simulink model "HyperscaleDataCenter"  (R2025b)
settings: Solver=VariableStepAuto  StartTime=0.0  StopTime=10  FixedStep=5e-5  RelTol=1e-4
PostLoadFcn:
  | HyperscaleDataCenterParam
values from neighbouring files (symbols this model uses):
  baseVoltageDC = 800    [DataCenterBBUParam.m]    (also in HyperscaleDataCenterParam.m; UPSBESSParam.m)
  bess_Ki = bess.controller.Ki    [SSTBESSParam.m]
  bess_Kp = bess.controller.Kp    [SSTBESSParam.m]
  droopGain = 0.02    [HyperscaleDataCenterParam.m]    (also in SSTBESSParam.m; UPSBESSParam.m)
  peakShavingPowerLimit = 800e3    (= 800000)    [HyperscaleDataCenterParam.m]
  powerTau = 0.005    [HyperscaleDataCenterParam.m]
  Prated_batt = 40e3    (= 40000)    [HyperscaleDataCenterParam.m]
  tauPS = 0.1    [HyperscaleDataCenterParam.m]
  Ts = 50e-6    (= 5e-05)    [BBUParam.m]    (also in DataCenterBBUParam.m; HyperscaleDataCenterParam.m)
  Ts_PS = 1e-3    (= 0.001)    [HyperscaleDataCenterParam.m]
undefined symbols (not defined in the file or in its folder): bbu, DiscIntNeverNeededParam, dspblkCoreblockFVToolHelper, ee_sli_rtmsupport, gcbh, grid, rack, sst, ups
libraries: fl_lib x80, nesl_utility x42, datacenter_lib x20, ee_lib x17, simulink x10, eeGeneralControl x9, slpidlib x6, microgridRenewables_lib x4, eeTransforms x4, batteryecm_lib x3, eeSinusoidalMeasurementV2 x2, simulink_extras x1
(part 5 of 5)

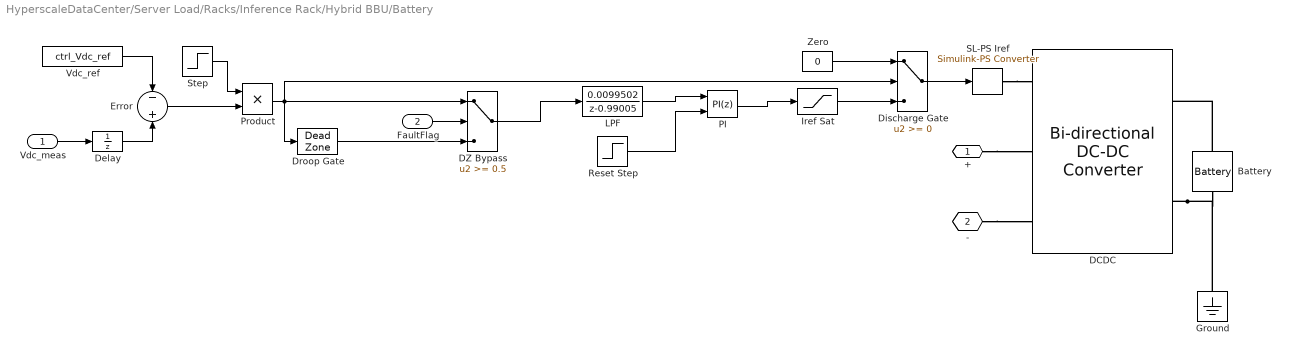
== system HyperscaleDataCenter/Server Load/Racks/Inference Rack/Hybrid BBU/Battery ==
  Vdc_meas : Inport
  FaultFlag : Inport  Port=2
  Battery : batteryecm_lib/Battery  Vnom=800 V  prm_dir=simscape.enum.battery.prm_dir.disabled  R1_dis=0.002 Ohm  R1_ch=0.002 Ohm  R1=0.004 Ohm  prm_AH=simscape.enum.battery.prm_AH.infinite  AH=50 A*hr  V1=11.5 V  AH1=25 A*hr  prm_R2=simscape.enum.battery.prm_R2.disabled  R2=2000 Ohm  Tmeas=298.15 K  charge_measurement_port=simscape.enum.battery.enable.no  prm_dyn=simscape.enum.battery.prm_dyn.off  Rp1=0.001 Ohm  tau1=30 s  Rp2=0.001 Ohm  tau2=30 s  Rp3=0.001 Ohm  tau3=30 s  Rp4=0.001 Ohm  tau4=30 s  Rp5=0.001 Ohm  tau5=30 s  prm_fade=simscape.enum.battery.prm_fade.disabled  N_fade=100  AH_fade=45 A*hr  R1_fade=2.02 Ohm  R1_ch_fade=2.02 Ohm  V1_fade=10.35 V  prm_age=simscape.enum.battery.prm_age.disabled  prm_age_OCV=simscape.enum.battery.prm_age_OCV.OCV  OCV_age=0.9  SOC_age=60  Tmeas_age=298.15 K  delta_time_age_vec=[0] d  temperature_age_vec=[273] K  OCV_scaling_age=2.2134e6  OCV_offset_age=1.632e6  temp_exp_age=0.515833569 V  t_exp_age=0.75  Vnom_T2=12 V  R1_T2=2.2 Ohm  R1_T2_dis=2.2 Ohm  R1_T2_ch=2.2 Ohm  V1_T2=11.4 V  R2_T2=2200 Ohm  Rp1_T2=0.005 Ohm  tau1_T2=30 s  Rp2_T2=0.005 Ohm  tau2_T2=30 s  Rp3_T2=0.005 Ohm  tau3_T2=30 s  Rp4_T2=0.005 Ohm  tau4_T2=30 s  Rp5_T2=0.005 Ohm  tau5_T2=30 s  Tmeas2=273.15 K  thermal_port=simscape.enum.thermaleffects.omit  thermal_mass=30000 J/K  i_specify=off  i_priority=None  i=0 A  i_nominal_specify=off  i_nominal_value=1  i_nominal_unit=A  v_specify=on  v_priority=None  v=800 V  v_nominal_specify=off  v_nominal_value=1  v_nominal_unit=V  charge_specify=off  charge_priority=None  charge=50 A*hr  charge_nominal_specify=off  charge_nominal_value=1  charge_nominal_unit=A*hr  num_cycles_specify=off  num_cycles_priority=High  num_cycles=0  num_cycles_nominal_specify=off  num_cycles_nominal_value=1  num_cycles_nominal_unit=1  temperature_specify=off  temperature_priority=High  temperature=298.15 K  temperature_nominal_specify=off  temperature_nominal_value=1  temperature_nominal_unit=K
  DCDC : microgridRenewables_lib/Bi-directional DC-DC Converter  efficiency_option=ee.enum.converters.efficiency.constant  efficiency_fixed=100  i_vec=[0, 2, 5] A  efficiency_vec=[90, 95, 98]  iL_specify=off  iL_priority=High  iL=0 A  iL_nominal_specify=off  iL_nominal_value=1  iL_nominal_unit=A  vc_specify=off  vc_priority=High  vc=0 V  vc_nominal_specify=off  vc_nominal_value=1  vc_nominal_unit=V  i1_specify=on  i1_priority=Low  i1=0 A  i1_nominal_specify=off  i1_nominal_value=1  i1_nominal_unit=A  i2_specify=on  i2_priority=Low  i2=0 A  i2_nominal_specify=off  i2_nominal_value=1  i2_nominal_unit=A  v1_specify=off  v1_priority=None  v1=0 V  v1_nominal_specify=off  v1_nominal_value=1  v1_nominal_unit=V  v2_specify=off  v2_priority=High  v2=800 V  v2_nominal_specify=off  v2_nominal_value=1  v2_nominal_unit=V
      settings: InternalSimscapePortConfiguration="{\"Bottom\":[],\"Left\":[{\"id\":\"Iref\",\"label\":\"Iref\",\"type\":\"input\"},{\"id\":\"p1\",\"label\":\"1+\",\"type\":\"foundation.electrical.electrical\"},{\"id\":\"n1\",\"label\":\"1-\",\"type\":\"foundation.electrical.electrical\"}],\"Right\":[{\"id\":\"p2\",\"label\":\"2+\",\"type\":\"foundation.electrical.electrical\"},{\"id\":\"n2\",\"label\":\"2-\",\"type\":\"foundation.electrical.electrical\"}],\"Top\":[]}"
  DZ Bypass : Switch  Threshold=0.5  SaturateOnIntegerOverflow=off  InputSameDT=off
  Delay : UnitDelay  InitialCondition=800  SampleTime=ctrl_Ts
  Discharge Gate : Switch  SaturateOnIntegerOverflow=off  InputSameDT=off
  Droop Gate : DeadZone  LowerValue=-60  UpperValue=60
  Error : Sum  Inputs=-+
  Ground : fl_lib/Electrical/Electrical Elements/Electrical Reference
  Iref Sat : Saturate  UpperLimit=0  LowerLimit=-10000
  LPF : DiscreteTransferFcn  Numerator=[0.0099502]  Denominator=[1 -0.99005]
  PI : slpidlib/PID Controller  Controller=PI  Form=Parallel  TimeDomain=Discrete-time  UseExternalTs=off  SampleTime=ctrl_Ts  IntegratorMethod=Forward Euler  FilterMethod=Forward Euler  ControllerParametersSource=internal  P=batt_Kp_ctrl  I=batt_Ki_ctrl  UseKiTs=off  D=0  UseExternalDerivativeSource=off  N=100  UseFilter=on  TunerSelectOption=Transfer Function Based (PID Tuner App)  InitialConditionSource=internal  InitialConditionForIntegrator=0  InitialConditionForFilter=0  DifferentiatorICPrevScaledInput=0  ExternalReset=rising  TrackingMode=off  Kt=1  LimitOutput=on  SatLimitsSource=internal  UpperSaturationLimit=0  LowerSaturationLimit=-batt_Imax  LinearizeAsGain=off  AntiWindupMode=clamping  Kb=1  LimitIntegrator=off  UpperIntegratorSaturationLimit=inf  LowerIntegratorSaturationLimit=-inf  POutMin=[]  POutMax=[]  IOutMin=[]  IOutMax=[]  DOutMin=[]  DOutMax=[]  NOutMin=[]  NOutMax=[]  SumOutMin=[]  SumOutMax=[]  SaturationOutMin=[]  SaturationOutMax=[]  PParamMin=[]  PParamMax=[]  IParamMin=[]  IParamMax=[]  DParamMin=[]  DParamMax=[]  NParamMin=[]  NParamMax=[]  KbParamMin=[]  KbParamMax=[]  KtParamMin=[]  KtParamMax=[]  KbOutMin=[]  KbOutMax=[]  KtOutMin=[]  KtOutMax=[]  IntegratorOutMin=[]  IntegratorOutMax=[]  FilterOutMin=[]  FilterOutMax=[]  SumI1OutMin=[]  SumI1OutMax=[]  SumI2OutMin=[]  SumI2OutMax=[]  SumI3OutMin=[]  SumI3OutMax=[]  SumI4OutMin=[]  SumI4OutMax=[]  SumDOutMin=[]  SumDOutMax=[]  DifferentiatorOutMin=[]  DifferentiatorOutMax=[]  FilterDiffOutCoefMin=[]  FilterDiffOutCoefMax=[]  ReciprocalOutMin=[]  ReciprocalOutMax=[]  SumDenOutMin=[]  SumDenOutMax=[]  SumNumOutMin=[]  SumNumOutMax=[]  DivideOutMin=[]  DivideOutMax=[]  UdiffTsProdOutMin=[]  UdiffTsProdOutMax=[]  NTsProdOutMin=[]  NTsProdOutMax=[]  UintegralTsProdOutMin=[]  UintegralTsProdOutMax=[]  UngainTsProdOutMin=[]  UngainTsProdOutMax=[]  ClampingZeroOutDataTypeStr=Inherit: Inherit via back propagation  ClampingZeroOutMin=[]  ClampingZeroOutMax=[]  FilterDenConstantOutDataTypeStr=Inherit: Inherit via back propagation  FilterDenConstantOutMin=[]  FilterDenConstantOutMax=[]  PCopyOutDataTypeStr=Inherit: Inherit via back propagation  PCopyOutMin=[]  PCopyOutMax=[]  NCopyOutDataTypeStr=Inherit: Inherit via back propagation  NCopyOutMin=[]  NCopyOutMax=[]  IntegratorContinuousStateAttributes=''  IntegratorStateMustResolveToSignalObject=off  IntegratorRTWStateStorageClass=Auto  FilterContinuousStateAttributes=''  FilterStateMustResolveToSignalObject=off  FilterRTWStateStorageClass=Auto  ParallelPVariant=InternalParameters  IdealPVariant=Disabled  IVariant=InternalParameters  DVariant=Disabled  IntegratorVariant=Discrete  SatVariant=Enabled  AWVariant=DiscClampingParallel  PCopyVariant=Disabled  TRVariant=Disabled  FdbkBlocksVariant=Forward  IdealPFdbkVariant=Disabled  SatFdbkVariant=Disabled  DerivativeFilterVariant=Disabled  NVariant=Disabled  NCopyVariant=Disabled_SignalSpec  FilterICVariant=Disabled  IntegratorICVariant=InternalICs  ExternalResetVariant=ExternalReset  TRSumVariant=Passthrough  SumFdbkVariant=Disabled  SumVariant=Sum_PI  TsampFilterVariant=InternalTs  TsampNgainVariant=Passthrough  TsampIntegralVariant=Disabled_SignalSpec  ExternalSaturationOutDataTypeStr=Inherit: Same as second input  DerivativeSourceVariant=Disabled  PreIntVariant=InternalPreInt
      settings: LibrarySourceBlock=simulink/Discrete/Discrete PID Controller
  Product : Product
  Reset Step : Step  Time=0.5  SampleTime=0
  SL-PS Iref : nesl_utility/Simulink-PS Converter  PhysicalDomain=network_engine_domain  SubClassName=ps_input  LeftPortType=input  RightPortType=output  PseudoPeriodic=off  Frequencies=[]  NoiseDistribution=none  NoiseParameters=[]  Unit=1  AffineConversion=off  FilteringAndDerivatives=filter  SimscapeFilterOrder=1  InputFilterTimeConstant=5e-05  UdotUserProvided=0
  Step : Step  Time=0  SampleTime=0
  Vdc_ref : Constant  Value=ctrl_Vdc_ref
  Zero : Constant  Value=0
  + : PMIOPort  Side=Left
  - : PMIOPort  Port=2  Side=Left
  wires:
  Vdc_ref/1 -> Error/1
  Delay/1 -> Error/2
  LPF/1 -> PI/1
  PI/1 -> Iref Sat/1
  Vdc_meas/1 -> Delay/1
  FaultFlag/1 -> DZ Bypass/2
  Droop Gate/1 -> DZ Bypass/3
  DZ Bypass/1 -> LPF/1
  Zero/1 -> Discharge Gate/1
  Iref Sat/1 -> Discharge Gate/3
  Discharge Gate/1 -> SL-PS Iref/1
  Step/1 -> Product/1
  Error/1 -> Product/2
  Product/1 -> Discharge Gate/2, Droop Gate/1, DZ Bypass/1
  Reset Step/1 -> PI/2
  connections:
  +/RConn1 -- DCDC/LConn2
  DCDC/RConn2 -- Ground/LConn1 -- Battery/RConn1
  Battery/LConn1 -- DCDC/RConn1
  -/RConn1 -- DCDC/LConn3
  SL-PS Iref/RConn1 -- DCDC/LConn1

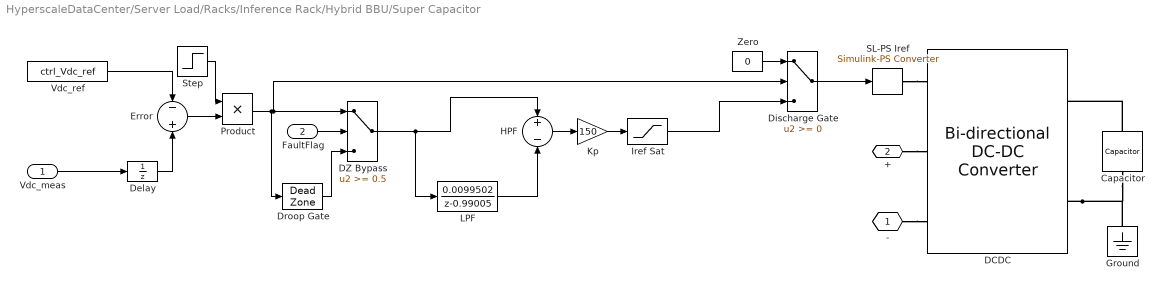
== system HyperscaleDataCenter/Server Load/Racks/Inference Rack/Hybrid BBU/Super Capacitor ==
  Vdc_meas : Inport
  FaultFlag : Inport  Port=2
  Capacitor : fl_lib/Electrical/Electrical Elements/Capacitor  c=5 F  r=1e-06 Ohm  g=0 1/Ohm  i_specify=off  i_priority=None  i=0 A  i_nominal_specify=off  i_nominal_value=1  i_nominal_unit=A  v_specify=on  v_priority=None  v=800 V  v_nominal_specify=off  v_nominal_value=1  v_nominal_unit=V  vc_specify=on  vc_priority=None  vc=800 V  vc_nominal_specify=off  vc_nominal_value=1  vc_nominal_unit=V
  DCDC : microgridRenewables_lib/Bi-directional DC-DC Converter  efficiency_option=ee.enum.converters.efficiency.constant  efficiency_fixed=100  i_vec=[0, 2, 5] A  efficiency_vec=[90, 95, 98]  iL_specify=off  iL_priority=High  iL=0 A  iL_nominal_specify=off  iL_nominal_value=1  iL_nominal_unit=A  vc_specify=off  vc_priority=High  vc=0 V  vc_nominal_specify=off  vc_nominal_value=1  vc_nominal_unit=V  i1_specify=on  i1_priority=Low  i1=0 A  i1_nominal_specify=off  i1_nominal_value=1  i1_nominal_unit=A  i2_specify=on  i2_priority=Low  i2=0 A  i2_nominal_specify=off  i2_nominal_value=1  i2_nominal_unit=A  v1_specify=off  v1_priority=None  v1=0 V  v1_nominal_specify=off  v1_nominal_value=1  v1_nominal_unit=V  v2_specify=off  v2_priority=High  v2=800 V  v2_nominal_specify=off  v2_nominal_value=1  v2_nominal_unit=V
      settings: InternalSimscapePortConfiguration="{\"Bottom\":[],\"Left\":[{\"id\":\"Iref\",\"label\":\"Iref\",\"type\":\"input\"},{\"id\":\"p1\",\"label\":\"1+\",\"type\":\"foundation.electrical.electrical\"},{\"id\":\"n1\",\"label\":\"1-\",\"type\":\"foundation.electrical.electrical\"}],\"Right\":[{\"id\":\"p2\",\"label\":\"2+\",\"type\":\"foundation.electrical.electrical\"},{\"id\":\"n2\",\"label\":\"2-\",\"type\":\"foundation.electrical.electrical\"}],\"Top\":[]}"
  DZ Bypass : Switch  Threshold=0.5  SaturateOnIntegerOverflow=off  InputSameDT=off
  Delay : UnitDelay  InitialCondition=800  SampleTime=ctrl_Ts
  Discharge Gate : Switch  SaturateOnIntegerOverflow=off  InputSameDT=off
  Droop Gate : DeadZone  LowerValue=-60  UpperValue=60
  Error : Sum  Inputs=-+
  Ground : fl_lib/Electrical/Electrical Elements/Electrical Reference
  HPF : Sum  Inputs=+-
  Iref Sat : Saturate  UpperLimit=0  LowerLimit=-12000
  Kp : Gain  Gain=150
  LPF : DiscreteTransferFcn  LoadFcn=dspblkCoreblockFVToolHelper(gcbh,'load');  Numerator=[0.0099502]  Denominator=[1 -0.99005]
      settings: CopyFcn=dspblkCoreblockFVToolHelper(gcbh,'copy');  DeleteFcn=dspblkCoreblockFVToolHelper(gcbh,'close');  ModelCloseFcn=dspblkCoreblockFVToolHelper(gcbh,'close');  PreSaveFcn=dspblkCoreblockFVToolHelper(gcbh,'presave');  PostSaveFcn=dspblkCoreblockFVToolHelper(gcbh,'postsave');  CloseFcn=dspblkCoreblockFVToolHelper(gcbh,'close');
  Product : Product
  SL-PS Iref : nesl_utility/Simulink-PS Converter  PhysicalDomain=network_engine_domain  SubClassName=ps_input  LeftPortType=input  RightPortType=output  PseudoPeriodic=off  Frequencies=[]  NoiseDistribution=none  NoiseParameters=[]  Unit=1  AffineConversion=off  FilteringAndDerivatives=filter  SimscapeFilterOrder=1  InputFilterTimeConstant=1e-05  UdotUserProvided=0
  Step : Step  Time=0  SampleTime=0
  Vdc_ref : Constant  Value=ctrl_Vdc_ref
  Zero : Constant  Value=0
  - : PMIOPort  Side=Left
  + : PMIOPort  Port=2  Side=Left
  wires:
  Vdc_ref/1 -> Error/1
  Delay/1 -> Error/2
  Kp/1 -> Iref Sat/1
  Droop Gate/1 -> DZ Bypass/3
  LPF/1 -> HPF/2
  HPF/1 -> Kp/1
  Vdc_meas/1 -> Delay/1
  FaultFlag/1 -> DZ Bypass/2
  DZ Bypass/1 -> HPF/1, LPF/1
  Zero/1 -> Discharge Gate/1
  Iref Sat/1 -> Discharge Gate/3
  Discharge Gate/1 -> SL-PS Iref/1
  Step/1 -> Product/1
  Error/1 -> Product/2
  Product/1 -> Droop Gate/1, Discharge Gate/2, DZ Bypass/1
  connections:
  +/RConn1 -- DCDC/LConn2
  DCDC/RConn2 -- Ground/LConn1 -- Capacitor/RConn1
  Capacitor/LConn1 -- DCDC/RConn1
  -/RConn1 -- DCDC/LConn3
  SL-PS Iref/RConn1 -- DCDC/LConn1

== system HyperscaleDataCenter/Server Load/Racks/Inference Rack/PDU Racks/Server Tray ==
  AmbCPU : fl_lib/Thermal/Thermal Elements/Convective Heat Transfer  thermal_type=foundation.enum.constant_variable.constant  area=cpuSurfArea*nCPU m^2  heat_tr_coeff=htc W/(K*m^2)  min_heat_tr_coeff=1e-3 W/(K*m^2)  T_specify=off  T_priority=None  T=0 K  T_nominal_specify=off  T_nominal_value=1  T_nominal_unit=K  Q_specify=off  Q_priority=None  Q=0 W  Q_nominal_specify=off  Q_nominal_value=1  Q_nominal_unit=W
  AmbGPU : fl_lib/Thermal/Thermal Elements/Convective Heat Transfer  thermal_type=foundation.enum.constant_variable.constant  area=gpuSurfArea*nGPU m^2  heat_tr_coeff=htc W/(K*m^2)  min_heat_tr_coeff=1e-3 W/(K*m^2)  T_specify=off  T_priority=None  T=0 K  T_nominal_specify=off  T_nominal_value=1  T_nominal_unit=K  Q_specify=off  Q_priority=None  Q=0 W  Q_nominal_specify=off  Q_nominal_value=1  Q_nominal_unit=W
  PS Add : fl_lib/Physical Signals/Functions/PS Add
  Server Chip CPU : datacenter_lib/Server Chip  processorType=ProcessorType.CPU  numGPUs=4  numCPUs=nCPU  gpuTDP=1200 W  gpuIdlePower=300 W  gpuPowerExponent=1.4  hbmPowPerGPU=80 W  hbmUtilizationFrac=0.7  cpuTDP=cpuTDPperSocket W  cpuIdlePower=cpuIdlePower W  cpuPowerExponent=cpuExponent  PleakageCoeff=cpuLeakage W/K  chipTnominal=cpuNominalDieT K  chipCth=cpuDieThermalC J/K  T_specify=on  T_priority=None  T=initialT K  T_nominal_specify=off  T_nominal_value=1  T_nominal_unit=K  Q_specify=off  Q_priority=None  Q=0 W  Q_nominal_specify=off  Q_nominal_value=1  Q_nominal_unit=W
      settings: InternalSimscapePortConfiguration="{\"Bottom\":[{\"id\":\"H\",\"label\":\"H\",\"type\":\"foundation.thermal.thermal\"}],\"Left\":[{\"id\":\"U\",\"label\":\"U\",\"type\":\"input\"}],\"Right\":[{\"id\":\"Pow\",\"label\":\"P\",\"type\":\"output\"},{\"id\":\"Tchip\",\"label\":\"T\",\"type\":\"output\"}],\"Top\":[]}"
  Server Chip GPU : datacenter_lib/Server Chip  processorType=ProcessorType.GPU  numGPUs=nGPU  numCPUs=nCPU  gpuTDP=gpuTDPperDie W  gpuIdlePower=gpuIdlePower W  gpuPowerExponent=gpuExponent  hbmPowPerGPU=gpuHBMpower W  hbmUtilizationFrac=gpuHBMutil  cpuTDP=cpuTDPperSocket W  cpuIdlePower=cpuIdlePower W  cpuPowerExponent=1.1  PleakageCoeff=gpuLeakage W/K  chipTnominal=gpuNominalDieT K  chipCth=gpuDieThermalC J/K  T_specify=on  T_priority=None  T=initialT K  T_nominal_specify=off  T_nominal_value=1  T_nominal_unit=K  Q_specify=off  Q_priority=None  Q=0 W  Q_nominal_specify=off  Q_nominal_value=1  Q_nominal_unit=W
      settings: InternalSimscapePortConfiguration="{\"Bottom\":[{\"id\":\"H\",\"label\":\"H\",\"type\":\"foundation.thermal.thermal\"}],\"Left\":[{\"id\":\"U\",\"label\":\"U\",\"type\":\"input\"}],\"Right\":[{\"id\":\"Pow\",\"label\":\"P\",\"type\":\"output\"},{\"id\":\"Tchip\",\"label\":\"T\",\"type\":\"output\"}],\"Top\":[]}"
  TR_CPU_Amb : fl_lib/Thermal/Thermal Elements/Thermal Resistance  resistance=cpuAmbientR/nGPU K/W  T_specify=off  T_priority=None  T=0 K  T_nominal_specify=off  T_nominal_value=1  T_nominal_unit=K  Q_specify=off  Q_priority=None  Q=0 W  Q_nominal_specify=off  Q_nominal_value=1  Q_nominal_unit=W
  TR_CPU_substrate : fl_lib/Thermal/Thermal Elements/Thermal Resistance  resistance=cpuHeatSinkR/nGPU K/W  T_specify=off  T_priority=None  T=0 K  T_nominal_specify=off  T_nominal_value=1  T_nominal_unit=K  Q_specify=off  Q_priority=None  Q=0 W  Q_nominal_specify=off  Q_nominal_value=1  Q_nominal_unit=W
  TR_GPU_Amb : fl_lib/Thermal/Thermal Elements/Thermal Resistance  resistance=gpuAmbientR/nGPU K/W  T_specify=off  T_priority=None  T=0 K  T_nominal_specify=off  T_nominal_value=1  T_nominal_unit=K  Q_specify=off  Q_priority=None  Q=0 W  Q_nominal_specify=off  Q_nominal_value=1  Q_nominal_unit=W
  TR_GPU_substrate : fl_lib/Thermal/Thermal Elements/Thermal Resistance  resistance=gpuHeatSinkR/nGPU K/W  T_specify=off  T_priority=None  T=0 K  T_nominal_specify=off  T_nominal_value=1  T_nominal_unit=K  Q_specify=off  Q_priority=None  Q=0 W  Q_nominal_specify=off  Q_nominal_value=1  Q_nominal_unit=W
  TR_Tray_Amb : fl_lib/Thermal/Thermal Elements/Thermal Resistance  resistance=trayThermalR K/W  T_specify=off  T_priority=None  T=0 K  T_nominal_specify=off  T_nominal_value=1  T_nominal_unit=K  Q_specify=off  Q_priority=None  Q=0 W  Q_nominal_specify=off  Q_nominal_value=1  Q_nominal_unit=W
  Tray Thermal Mass : fl_lib/Thermal/Thermal Elements/Thermal Mass  mass_type=foundation.enum.constant_variable.constant  mass=trayMass kg  sp_heat=trayCp J/(K*kg)  mass_min=1e-6 kg  num_ports=foundation.enum.numPorts2.two  m_specify=off  m_priority=None  m=1 kg  m_nominal_specify=off  m_nominal_value=1  m_nominal_unit=kg  T_specify=on  T_priority=None  T=initialT K  T_nominal_specify=off  T_nominal_value=1  T_nominal_unit=K  Q_specify=off  Q_priority=None  Q=0 W  Q_nominal_specify=off  Q_nominal_value=1  Q_nominal_unit=W
      settings: InternalSimscapePortConfiguration="{\"Bottom\":[],\"Left\":[{\"id\":\"M\",\"label\":\"\",\"type\":\"foundation.thermal.thermal\"}],\"Right\":[{\"id\":\"N\",\"label\":\"\",\"type\":\"foundation.thermal.thermal\"}],\"Top\":[]}"
  U_gpu : PMIOPort  Side=Left
  U_cpu : PMIOPort  Port=2  Side=Left
  P : PMIOPort  Port=3  Side=Right
  T_gpu : PMIOPort  Port=4  Side=Right
  T_cpu : PMIOPort  Port=5  Side=Right
  Hc : PMIOPort  Port=6  Side=Right
  Ha : PMIOPort  Port=7  Side=Left
  connections:
  AmbCPU/LConn1 -- TR_CPU_Amb/RConn1
  PS Add/LConn2 -- Server Chip CPU/RConn1
  PS Add/LConn1 -- Server Chip GPU/RConn1
  P/RConn1 -- PS Add/RConn1
  Ha/RConn1 -- AmbGPU/RConn1 -- AmbCPU/RConn1
  AmbGPU/LConn1 -- TR_GPU_Amb/LConn1
  TR_Tray_Amb/RConn1 -- Hc/RConn1
  Server Chip CPU/RConn2 -- T_cpu/RConn1
  Server Chip CPU/LConn1 -- U_cpu/RConn1
  Server Chip GPU/LConn1 -- U_gpu/RConn1
  TR_Tray_Amb/LConn1 -- Tray Thermal Mass/RConn1
  TR_GPU_substrate/LConn1 -- Server Chip GPU/RConn3 -- TR_GPU_Amb/RConn1
  Server Chip CPU/RConn3 -- TR_CPU_Amb/LConn1 -- TR_CPU_substrate/LConn1
  Server Chip GPU/RConn2 -- T_gpu/RConn1
  TR_CPU_substrate/RConn1 -- TR_GPU_substrate/RConn1 -- Tray Thermal Mass/LConn1

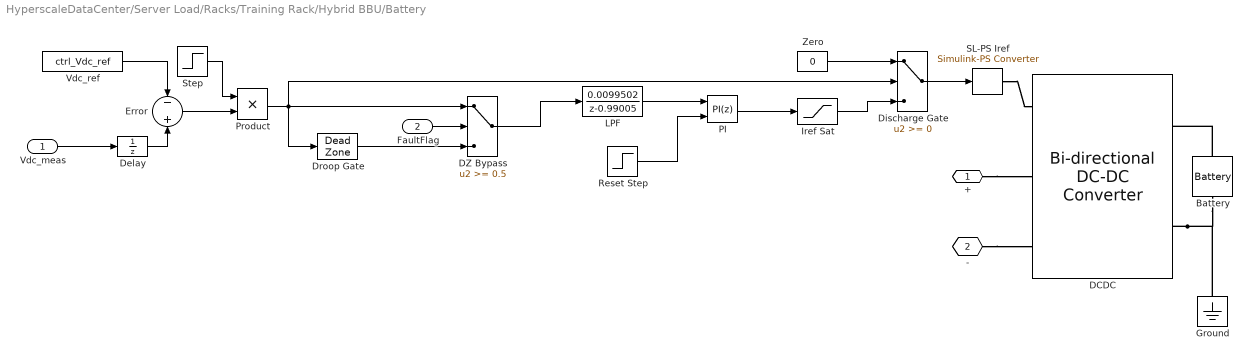
== system HyperscaleDataCenter/Server Load/Racks/Training Rack/Hybrid BBU/Battery ==
  Vdc_meas : Inport
  FaultFlag : Inport  Port=2
  Battery : batteryecm_lib/Battery  Vnom=800 V  prm_dir=simscape.enum.battery.prm_dir.disabled  R1_dis=0.002 Ohm  R1_ch=0.002 Ohm  R1=0.004 Ohm  prm_AH=simscape.enum.battery.prm_AH.infinite  AH=50 A*hr  V1=11.5 V  AH1=25 A*hr  prm_R2=simscape.enum.battery.prm_R2.disabled  R2=2000 Ohm  Tmeas=298.15 K  charge_measurement_port=simscape.enum.battery.enable.no  prm_dyn=simscape.enum.battery.prm_dyn.off  Rp1=0.001 Ohm  tau1=30 s  Rp2=0.001 Ohm  tau2=30 s  Rp3=0.001 Ohm  tau3=30 s  Rp4=0.001 Ohm  tau4=30 s  Rp5=0.001 Ohm  tau5=30 s  prm_fade=simscape.enum.battery.prm_fade.disabled  N_fade=100  AH_fade=45 A*hr  R1_fade=2.02 Ohm  R1_ch_fade=2.02 Ohm  V1_fade=10.35 V  prm_age=simscape.enum.battery.prm_age.disabled  prm_age_OCV=simscape.enum.battery.prm_age_OCV.OCV  OCV_age=0.9  SOC_age=60  Tmeas_age=298.15 K  delta_time_age_vec=[0] d  temperature_age_vec=[273] K  OCV_scaling_age=2.2134e6  OCV_offset_age=1.632e6  temp_exp_age=0.515833569 V  t_exp_age=0.75  Vnom_T2=12 V  R1_T2=2.2 Ohm  R1_T2_dis=2.2 Ohm  R1_T2_ch=2.2 Ohm  V1_T2=11.4 V  R2_T2=2200 Ohm  Rp1_T2=0.005 Ohm  tau1_T2=30 s  Rp2_T2=0.005 Ohm  tau2_T2=30 s  Rp3_T2=0.005 Ohm  tau3_T2=30 s  Rp4_T2=0.005 Ohm  tau4_T2=30 s  Rp5_T2=0.005 Ohm  tau5_T2=30 s  Tmeas2=273.15 K  thermal_port=simscape.enum.thermaleffects.omit  thermal_mass=30000 J/K  i_specify=off  i_priority=None  i=0 A  i_nominal_specify=off  i_nominal_value=1  i_nominal_unit=A  v_specify=on  v_priority=None  v=800 V  v_nominal_specify=off  v_nominal_value=1  v_nominal_unit=V  charge_specify=off  charge_priority=None  charge=50 A*hr  charge_nominal_specify=off  charge_nominal_value=1  charge_nominal_unit=A*hr  num_cycles_specify=off  num_cycles_priority=High  num_cycles=0  num_cycles_nominal_specify=off  num_cycles_nominal_value=1  num_cycles_nominal_unit=1  temperature_specify=off  temperature_priority=High  temperature=298.15 K  temperature_nominal_specify=off  temperature_nominal_value=1  temperature_nominal_unit=K
  DCDC : microgridRenewables_lib/Bi-directional DC-DC Converter  efficiency_option=ee.enum.converters.efficiency.constant  efficiency_fixed=100  i_vec=[0, 2, 5] A  efficiency_vec=[90, 95, 98]  iL_specify=off  iL_priority=High  iL=0 A  iL_nominal_specify=off  iL_nominal_value=1  iL_nominal_unit=A  vc_specify=off  vc_priority=High  vc=0 V  vc_nominal_specify=off  vc_nominal_value=1  vc_nominal_unit=V  i1_specify=on  i1_priority=Low  i1=0 A  i1_nominal_specify=off  i1_nominal_value=1  i1_nominal_unit=A  i2_specify=on  i2_priority=Low  i2=0 A  i2_nominal_specify=off  i2_nominal_value=1  i2_nominal_unit=A  v1_specify=off  v1_priority=None  v1=0 V  v1_nominal_specify=off  v1_nominal_value=1  v1_nominal_unit=V  v2_specify=off  v2_priority=High  v2=800 V  v2_nominal_specify=off  v2_nominal_value=1  v2_nominal_unit=V
      settings: InternalSimscapePortConfiguration="{\"Bottom\":[],\"Left\":[{\"id\":\"Iref\",\"label\":\"Iref\",\"type\":\"input\"},{\"id\":\"p1\",\"label\":\"1+\",\"type\":\"foundation.electrical.electrical\"},{\"id\":\"n1\",\"label\":\"1-\",\"type\":\"foundation.electrical.electrical\"}],\"Right\":[{\"id\":\"p2\",\"label\":\"2+\",\"type\":\"foundation.electrical.electrical\"},{\"id\":\"n2\",\"label\":\"2-\",\"type\":\"foundation.electrical.electrical\"}],\"Top\":[]}"
  DZ Bypass : Switch  Threshold=0.5  SaturateOnIntegerOverflow=off  InputSameDT=off
  Delay : UnitDelay  InitialCondition=800  SampleTime=ctrl_Ts
  Discharge Gate : Switch  SaturateOnIntegerOverflow=off  InputSameDT=off
  Droop Gate : DeadZone  LowerValue=-60  UpperValue=60
  Error : Sum  Inputs=-+
  Ground : fl_lib/Electrical/Electrical Elements/Electrical Reference
  Iref Sat : Saturate  UpperLimit=0  LowerLimit=-10000
  LPF : DiscreteTransferFcn  Numerator=[0.0099502]  Denominator=[1 -0.99005]
  PI : slpidlib/PID Controller  Controller=PI  Form=Parallel  TimeDomain=Discrete-time  UseExternalTs=off  SampleTime=ctrl_Ts  IntegratorMethod=Forward Euler  FilterMethod=Forward Euler  ControllerParametersSource=internal  P=batt_Kp_ctrl  I=batt_Ki_ctrl  UseKiTs=off  D=0  UseExternalDerivativeSource=off  N=100  UseFilter=on  TunerSelectOption=Transfer Function Based (PID Tuner App)  InitialConditionSource=internal  InitialConditionForIntegrator=0  InitialConditionForFilter=0  DifferentiatorICPrevScaledInput=0  ExternalReset=rising  TrackingMode=off  Kt=1  LimitOutput=on  SatLimitsSource=internal  UpperSaturationLimit=0  LowerSaturationLimit=-batt_Imax  LinearizeAsGain=off  AntiWindupMode=clamping  Kb=1  LimitIntegrator=off  UpperIntegratorSaturationLimit=inf  LowerIntegratorSaturationLimit=-inf  POutMin=[]  POutMax=[]  IOutMin=[]  IOutMax=[]  DOutMin=[]  DOutMax=[]  NOutMin=[]  NOutMax=[]  SumOutMin=[]  SumOutMax=[]  SaturationOutMin=[]  SaturationOutMax=[]  PParamMin=[]  PParamMax=[]  IParamMin=[]  IParamMax=[]  DParamMin=[]  DParamMax=[]  NParamMin=[]  NParamMax=[]  KbParamMin=[]  KbParamMax=[]  KtParamMin=[]  KtParamMax=[]  KbOutMin=[]  KbOutMax=[]  KtOutMin=[]  KtOutMax=[]  IntegratorOutMin=[]  IntegratorOutMax=[]  FilterOutMin=[]  FilterOutMax=[]  SumI1OutMin=[]  SumI1OutMax=[]  SumI2OutMin=[]  SumI2OutMax=[]  SumI3OutMin=[]  SumI3OutMax=[]  SumI4OutMin=[]  SumI4OutMax=[]  SumDOutMin=[]  SumDOutMax=[]  DifferentiatorOutMin=[]  DifferentiatorOutMax=[]  FilterDiffOutCoefMin=[]  FilterDiffOutCoefMax=[]  ReciprocalOutMin=[]  ReciprocalOutMax=[]  SumDenOutMin=[]  SumDenOutMax=[]  SumNumOutMin=[]  SumNumOutMax=[]  DivideOutMin=[]  DivideOutMax=[]  UdiffTsProdOutMin=[]  UdiffTsProdOutMax=[]  NTsProdOutMin=[]  NTsProdOutMax=[]  UintegralTsProdOutMin=[]  UintegralTsProdOutMax=[]  UngainTsProdOutMin=[]  UngainTsProdOutMax=[]  ClampingZeroOutDataTypeStr=Inherit: Inherit via back propagation  ClampingZeroOutMin=[]  ClampingZeroOutMax=[]  FilterDenConstantOutDataTypeStr=Inherit: Inherit via back propagation  FilterDenConstantOutMin=[]  FilterDenConstantOutMax=[]  PCopyOutDataTypeStr=Inherit: Inherit via back propagation  PCopyOutMin=[]  PCopyOutMax=[]  NCopyOutDataTypeStr=Inherit: Inherit via back propagation  NCopyOutMin=[]  NCopyOutMax=[]  IntegratorContinuousStateAttributes=''  IntegratorStateMustResolveToSignalObject=off  IntegratorRTWStateStorageClass=Auto  FilterContinuousStateAttributes=''  FilterStateMustResolveToSignalObject=off  FilterRTWStateStorageClass=Auto  ParallelPVariant=InternalParameters  IdealPVariant=Disabled  IVariant=InternalParameters  DVariant=Disabled  IntegratorVariant=Discrete  SatVariant=Enabled  AWVariant=DiscClampingParallel  PCopyVariant=Disabled  TRVariant=Disabled  FdbkBlocksVariant=Forward  IdealPFdbkVariant=Disabled  SatFdbkVariant=Disabled  DerivativeFilterVariant=Disabled  NVariant=Disabled  NCopyVariant=Disabled_SignalSpec  FilterICVariant=Disabled  IntegratorICVariant=InternalICs  ExternalResetVariant=ExternalReset  TRSumVariant=Passthrough  SumFdbkVariant=Disabled  SumVariant=Sum_PI  TsampFilterVariant=InternalTs  TsampNgainVariant=Passthrough  TsampIntegralVariant=Disabled_SignalSpec  ExternalSaturationOutDataTypeStr=Inherit: Same as second input  DerivativeSourceVariant=Disabled  PreIntVariant=InternalPreInt
      settings: LibrarySourceBlock=simulink/Discrete/Discrete PID Controller
  Product : Product
  Reset Step : Step  Time=0.5  SampleTime=0
  SL-PS Iref : nesl_utility/Simulink-PS Converter  PhysicalDomain=network_engine_domain  SubClassName=ps_input  LeftPortType=input  RightPortType=output  PseudoPeriodic=off  Frequencies=[]  NoiseDistribution=none  NoiseParameters=[]  Unit=1  AffineConversion=off  FilteringAndDerivatives=filter  SimscapeFilterOrder=1  InputFilterTimeConstant=5e-05  UdotUserProvided=0
  Step : Step  Time=0  SampleTime=0
  Vdc_ref : Constant  Value=ctrl_Vdc_ref
  Zero : Constant  Value=0
  + : PMIOPort  Side=Left
  - : PMIOPort  Port=2  Side=Left
  wires:
  Vdc_ref/1 -> Error/1
  Delay/1 -> Error/2
  LPF/1 -> PI/1
  PI/1 -> Iref Sat/1
  Vdc_meas/1 -> Delay/1
  FaultFlag/1 -> DZ Bypass/2
  Droop Gate/1 -> DZ Bypass/3
  DZ Bypass/1 -> LPF/1
  Zero/1 -> Discharge Gate/1
  Iref Sat/1 -> Discharge Gate/3
  Discharge Gate/1 -> SL-PS Iref/1
  Step/1 -> Product/1
  Error/1 -> Product/2
  Product/1 -> Discharge Gate/2, Droop Gate/1, DZ Bypass/1
  Reset Step/1 -> PI/2
  connections:
  +/RConn1 -- DCDC/LConn2
  DCDC/RConn2 -- Ground/LConn1 -- Battery/RConn1
  Battery/LConn1 -- DCDC/RConn1
  -/RConn1 -- DCDC/LConn3
  SL-PS Iref/RConn1 -- DCDC/LConn1

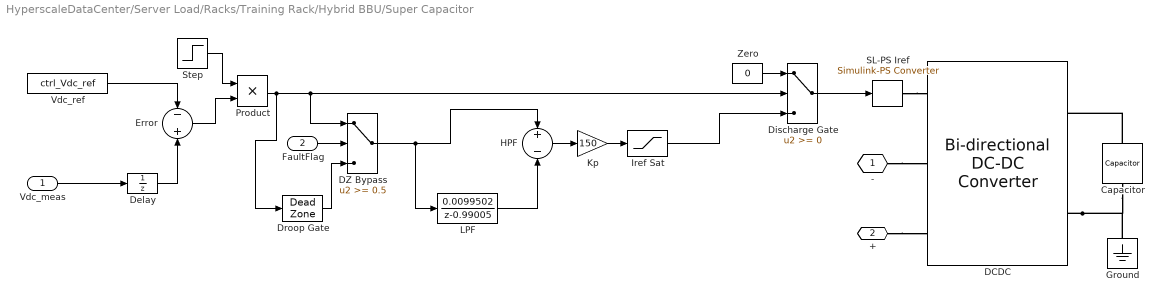
== system HyperscaleDataCenter/Server Load/Racks/Training Rack/Hybrid BBU/Super Capacitor ==
  Vdc_meas : Inport
  FaultFlag : Inport  Port=2
  Capacitor : fl_lib/Electrical/Electrical Elements/Capacitor  c=5 F  r=1e-06 Ohm  g=0 1/Ohm  i_specify=off  i_priority=None  i=0 A  i_nominal_specify=off  i_nominal_value=1  i_nominal_unit=A  v_specify=off  v_priority=None  v=0 V  v_nominal_specify=off  v_nominal_value=1  v_nominal_unit=V  vc_specify=on  vc_priority=None  vc=800 V  vc_nominal_specify=off  vc_nominal_value=1  vc_nominal_unit=V
  DCDC : microgridRenewables_lib/Bi-directional DC-DC Converter  efficiency_option=ee.enum.converters.efficiency.constant  efficiency_fixed=100  i_vec=[0, 2, 5] A  efficiency_vec=[90, 95, 98]  iL_specify=off  iL_priority=High  iL=0 A  iL_nominal_specify=off  iL_nominal_value=1  iL_nominal_unit=A  vc_specify=off  vc_priority=High  vc=0 V  vc_nominal_specify=off  vc_nominal_value=1  vc_nominal_unit=V  i1_specify=on  i1_priority=Low  i1=0 A  i1_nominal_specify=off  i1_nominal_value=1  i1_nominal_unit=A  i2_specify=on  i2_priority=Low  i2=0 A  i2_nominal_specify=off  i2_nominal_value=1  i2_nominal_unit=A  v1_specify=off  v1_priority=None  v1=0 V  v1_nominal_specify=off  v1_nominal_value=1  v1_nominal_unit=V  v2_specify=off  v2_priority=High  v2=800 V  v2_nominal_specify=off  v2_nominal_value=1  v2_nominal_unit=V
      settings: InternalSimscapePortConfiguration="{\"Bottom\":[],\"Left\":[{\"id\":\"Iref\",\"label\":\"Iref\",\"type\":\"input\"},{\"id\":\"p1\",\"label\":\"1+\",\"type\":\"foundation.electrical.electrical\"},{\"id\":\"n1\",\"label\":\"1-\",\"type\":\"foundation.electrical.electrical\"}],\"Right\":[{\"id\":\"p2\",\"label\":\"2+\",\"type\":\"foundation.electrical.electrical\"},{\"id\":\"n2\",\"label\":\"2-\",\"type\":\"foundation.electrical.electrical\"}],\"Top\":[]}"
  DZ Bypass : Switch  Threshold=0.5  SaturateOnIntegerOverflow=off  InputSameDT=off
  Delay : UnitDelay  InitialCondition=800  SampleTime=ctrl_Ts
  Discharge Gate : Switch  SaturateOnIntegerOverflow=off  InputSameDT=off
  Droop Gate : DeadZone  LowerValue=-60  UpperValue=60
  Error : Sum  Inputs=-+
  Ground : fl_lib/Electrical/Electrical Elements/Electrical Reference
  HPF : Sum  Inputs=+-
  Iref Sat : Saturate  UpperLimit=0  LowerLimit=-12000
  Kp : Gain  Gain=150
  LPF : DiscreteTransferFcn  LoadFcn=dspblkCoreblockFVToolHelper(gcbh,'load');  Numerator=[0.0099502]  Denominator=[1 -0.99005]
      settings: CopyFcn=dspblkCoreblockFVToolHelper(gcbh,'copy');  DeleteFcn=dspblkCoreblockFVToolHelper(gcbh,'close');  ModelCloseFcn=dspblkCoreblockFVToolHelper(gcbh,'close');  PreSaveFcn=dspblkCoreblockFVToolHelper(gcbh,'presave');  PostSaveFcn=dspblkCoreblockFVToolHelper(gcbh,'postsave');  CloseFcn=dspblkCoreblockFVToolHelper(gcbh,'close');
  Product : Product
  SL-PS Iref : nesl_utility/Simulink-PS Converter  PhysicalDomain=network_engine_domain  SubClassName=ps_input  LeftPortType=input  RightPortType=output  PseudoPeriodic=off  Frequencies=[]  NoiseDistribution=none  NoiseParameters=[]  Unit=1  AffineConversion=off  FilteringAndDerivatives=filter  SimscapeFilterOrder=1  InputFilterTimeConstant=1e-05  UdotUserProvided=0
  Step : Step  Time=0  SampleTime=0
  Vdc_ref : Constant  Value=ctrl_Vdc_ref
  Zero : Constant  Value=0
  - : PMIOPort  Side=Left
  + : PMIOPort  Port=2  Side=Left
  wires:
  Vdc_ref/1 -> Error/1
  Delay/1 -> Error/2
  Kp/1 -> Iref Sat/1
  Droop Gate/1 -> DZ Bypass/3
  LPF/1 -> HPF/2
  HPF/1 -> Kp/1
  Vdc_meas/1 -> Delay/1
  FaultFlag/1 -> DZ Bypass/2
  DZ Bypass/1 -> HPF/1, LPF/1
  Zero/1 -> Discharge Gate/1
  Iref Sat/1 -> Discharge Gate/3
  Discharge Gate/1 -> SL-PS Iref/1
  Step/1 -> Product/1
  Error/1 -> Product/2
  Product/1 -> Discharge Gate/2, DZ Bypass/1, Droop Gate/1
  connections:
  DCDC/RConn2 -- Ground/LConn1 -- Capacitor/RConn1
  Capacitor/LConn1 -- DCDC/RConn1
  SL-PS Iref/RConn1 -- DCDC/LConn1
  -/RConn1 -- DCDC/LConn2
  +/RConn1 -- DCDC/LConn3

== system HyperscaleDataCenter/Server Load/Racks/Training Rack/PDU Racks/Server Tray ==
  AmbCPU : fl_lib/Thermal/Thermal Elements/Convective Heat Transfer  thermal_type=foundation.enum.constant_variable.constant  area=cpuSurfArea*nCPU m^2  heat_tr_coeff=htc W/(K*m^2)  min_heat_tr_coeff=1e-3 W/(K*m^2)  T_specify=off  T_priority=None  T=0 K  T_nominal_specify=off  T_nominal_value=1  T_nominal_unit=K  Q_specify=off  Q_priority=None  Q=0 W  Q_nominal_specify=off  Q_nominal_value=1  Q_nominal_unit=W
  AmbGPU : fl_lib/Thermal/Thermal Elements/Convective Heat Transfer  thermal_type=foundation.enum.constant_variable.constant  area=gpuSurfArea*nGPU m^2  heat_tr_coeff=htc W/(K*m^2)  min_heat_tr_coeff=1e-3 W/(K*m^2)  T_specify=off  T_priority=None  T=0 K  T_nominal_specify=off  T_nominal_value=1  T_nominal_unit=K  Q_specify=off  Q_priority=None  Q=0 W  Q_nominal_specify=off  Q_nominal_value=1  Q_nominal_unit=W
  PS Add : fl_lib/Physical Signals/Functions/PS Add
  Server Chip CPU : datacenter_lib/Server Chip  processorType=ProcessorType.CPU  numGPUs=4  numCPUs=nCPU  gpuTDP=1200 W  gpuIdlePower=300 W  gpuPowerExponent=1.4  hbmPowPerGPU=80 W  hbmUtilizationFrac=0.7  cpuTDP=cpuTDPperSocket W  cpuIdlePower=cpuIdlePower W  cpuPowerExponent=cpuExponent  PleakageCoeff=cpuLeakage W/K  chipTnominal=cpuNominalDieT K  chipCth=cpuDieThermalC J/K  T_specify=on  T_priority=None  T=initialT K  T_nominal_specify=off  T_nominal_value=1  T_nominal_unit=K  Q_specify=off  Q_priority=None  Q=0 W  Q_nominal_specify=off  Q_nominal_value=1  Q_nominal_unit=W
      settings: InternalSimscapePortConfiguration="{\"Bottom\":[{\"id\":\"H\",\"label\":\"H\",\"type\":\"foundation.thermal.thermal\"}],\"Left\":[{\"id\":\"U\",\"label\":\"U\",\"type\":\"input\"}],\"Right\":[{\"id\":\"Pow\",\"label\":\"P\",\"type\":\"output\"},{\"id\":\"Tchip\",\"label\":\"T\",\"type\":\"output\"}],\"Top\":[]}"
  Server Chip GPU : datacenter_lib/Server Chip  processorType=ProcessorType.GPU  numGPUs=nGPU  numCPUs=nCPU  gpuTDP=gpuTDPperDie W  gpuIdlePower=gpuIdlePower W  gpuPowerExponent=gpuExponent  hbmPowPerGPU=gpuHBMpower W  hbmUtilizationFrac=gpuHBMutil  cpuTDP=cpuTDPperSocket W  cpuIdlePower=cpuIdlePower W  cpuPowerExponent=1.1  PleakageCoeff=gpuLeakage W/K  chipTnominal=gpuNominalDieT K  chipCth=gpuDieThermalC J/K  T_specify=on  T_priority=None  T=initialT K  T_nominal_specify=off  T_nominal_value=1  T_nominal_unit=K  Q_specify=off  Q_priority=None  Q=0 W  Q_nominal_specify=off  Q_nominal_value=1  Q_nominal_unit=W
      settings: InternalSimscapePortConfiguration="{\"Bottom\":[{\"id\":\"H\",\"label\":\"H\",\"type\":\"foundation.thermal.thermal\"}],\"Left\":[{\"id\":\"U\",\"label\":\"U\",\"type\":\"input\"}],\"Right\":[{\"id\":\"Pow\",\"label\":\"P\",\"type\":\"output\"},{\"id\":\"Tchip\",\"label\":\"T\",\"type\":\"output\"}],\"Top\":[]}"
  TR_CPU_Amb : fl_lib/Thermal/Thermal Elements/Thermal Resistance  resistance=cpuAmbientR/nGPU K/W  T_specify=off  T_priority=None  T=0 K  T_nominal_specify=off  T_nominal_value=1  T_nominal_unit=K  Q_specify=off  Q_priority=None  Q=0 W  Q_nominal_specify=off  Q_nominal_value=1  Q_nominal_unit=W
  TR_CPU_substrate : fl_lib/Thermal/Thermal Elements/Thermal Resistance  resistance=cpuHeatSinkR/nGPU K/W  T_specify=off  T_priority=None  T=0 K  T_nominal_specify=off  T_nominal_value=1  T_nominal_unit=K  Q_specify=off  Q_priority=None  Q=0 W  Q_nominal_specify=off  Q_nominal_value=1  Q_nominal_unit=W
  TR_GPU_Amb : fl_lib/Thermal/Thermal Elements/Thermal Resistance  resistance=gpuAmbientR/nGPU K/W  T_specify=off  T_priority=None  T=0 K  T_nominal_specify=off  T_nominal_value=1  T_nominal_unit=K  Q_specify=off  Q_priority=None  Q=0 W  Q_nominal_specify=off  Q_nominal_value=1  Q_nominal_unit=W
  TR_GPU_substrate : fl_lib/Thermal/Thermal Elements/Thermal Resistance  resistance=gpuHeatSinkR/nGPU K/W  T_specify=off  T_priority=None  T=0 K  T_nominal_specify=off  T_nominal_value=1  T_nominal_unit=K  Q_specify=off  Q_priority=None  Q=0 W  Q_nominal_specify=off  Q_nominal_value=1  Q_nominal_unit=W
  TR_Tray_Amb : fl_lib/Thermal/Thermal Elements/Thermal Resistance  resistance=trayThermalR K/W  T_specify=off  T_priority=None  T=0 K  T_nominal_specify=off  T_nominal_value=1  T_nominal_unit=K  Q_specify=off  Q_priority=None  Q=0 W  Q_nominal_specify=off  Q_nominal_value=1  Q_nominal_unit=W
  Tray Thermal Mass : fl_lib/Thermal/Thermal Elements/Thermal Mass  mass_type=foundation.enum.constant_variable.constant  mass=trayMass kg  sp_heat=trayCp J/(K*kg)  mass_min=1e-6 kg  num_ports=foundation.enum.numPorts2.two  m_specify=off  m_priority=None  m=1 kg  m_nominal_specify=off  m_nominal_value=1  m_nominal_unit=kg  T_specify=on  T_priority=None  T=initialT K  T_nominal_specify=off  T_nominal_value=1  T_nominal_unit=K  Q_specify=off  Q_priority=None  Q=0 W  Q_nominal_specify=off  Q_nominal_value=1  Q_nominal_unit=W
      settings: InternalSimscapePortConfiguration="{\"Bottom\":[],\"Left\":[{\"id\":\"M\",\"label\":\"\",\"type\":\"foundation.thermal.thermal\"}],\"Right\":[{\"id\":\"N\",\"label\":\"\",\"type\":\"foundation.thermal.thermal\"}],\"Top\":[]}"
  U_gpu : PMIOPort  Side=Left
  U_cpu : PMIOPort  Port=2  Side=Left
  P : PMIOPort  Port=3  Side=Right
  T_gpu : PMIOPort  Port=4  Side=Right
  T_cpu : PMIOPort  Port=5  Side=Right
  Hc : PMIOPort  Port=6  Side=Right
  Ha : PMIOPort  Port=7  Side=Left
  connections:
  AmbCPU/LConn1 -- TR_CPU_Amb/RConn1
  PS Add/LConn2 -- Server Chip CPU/RConn1
  PS Add/LConn1 -- Server Chip GPU/RConn1
  P/RConn1 -- PS Add/RConn1
  Ha/RConn1 -- AmbGPU/RConn1 -- AmbCPU/RConn1
  AmbGPU/LConn1 -- TR_GPU_Amb/LConn1
  TR_Tray_Amb/RConn1 -- Hc/RConn1
  Server Chip CPU/RConn2 -- T_cpu/RConn1
  Server Chip CPU/LConn1 -- U_cpu/RConn1
  Server Chip GPU/LConn1 -- U_gpu/RConn1
  TR_Tray_Amb/LConn1 -- Tray Thermal Mass/RConn1
  TR_GPU_substrate/LConn1 -- Server Chip GPU/RConn3 -- TR_GPU_Amb/RConn1
  Server Chip CPU/RConn3 -- TR_CPU_Amb/LConn1 -- TR_CPU_substrate/LConn1
  Server Chip GPU/RConn2 -- T_gpu/RConn1
  TR_CPU_substrate/RConn1 -- TR_GPU_substrate/RConn1 -- Tray Thermal Mass/LConn1

== system HyperscaleDataCenter/Solid State Transformer/PFC Rectifier Controller/Current Controller/Id and Iq Controller/Id Reference Selector ==
  Vmag : Inport
  AND1 : Logic  IconShape=distinctive  AllPortsSameDT=off  OutDataTypeStr=boolean
  Bias : Bias  Bias=0.01  SaturateOnIntegerOverflow=off
  Compare To Constant : simulink/Logic and Bit Operations/Compare To Constant  relop=>  const=0.5  OutDataTypeStr=boolean
  Compare To Constant2 : simulink/Logic and Bit Operations/Compare To Constant  relop=>  const=0.05  OutDataTypeStr=boolean
  Data Type Conversion : DataTypeConversion  SaturateOnIntegerOverflow=off  RndMeth=Floor
  Data Type Conversion1 : DataTypeConversion  OutDataTypeStr=double  SaturateOnIntegerOverflow=off  RndMeth=Floor
  Discrete-Time Integrator : DiscreteIntegrator  IntegratorMethod=Integration: Backward Euler  ExternalReset=falling  SampleTime=ups.sampleTime  LimitOutput=on  UpperSaturationLimit=0.6  LowerSaturationLimit=0  ICPrevOutput=DiscIntNeverNeededParam  ICPrevScaledInput=DiscIntNeverNeededParam
  Mode : Outport
  wires:
  Data Type Conversion/1 -> Mode/1
  Data Type Conversion1/1 -> Discrete-Time Integrator/2, Discrete-Time Integrator/1, AND1/1
  Discrete-Time Integrator/1 -> Compare To Constant2/1
  Compare To Constant2/1 -> AND1/2
  AND1/1 -> Data Type Conversion/1
  Compare To Constant/1 -> Data Type Conversion1/1
  Vmag/1 -> Bias/1
  Bias/1 -> Compare To Constant/1

== system HyperscaleDataCenter/Solid State Transformer/PFC Rectifier Controller/DC Voltage Controller and Current Reference/Voltage Controller/Voltage control ==
  e : Inport
  Reset : Inport  Port=2
  Discrete-Time Integrator : DiscreteIntegrator  IntegratorMethod=Integration: Backward Euler  ExternalReset=falling  SampleTime=ups.sampleTime  LimitOutput=on  UpperSaturationLimit=1  LowerSaturationLimit=0  ICPrevOutput=DiscIntNeverNeededParam  ICPrevScaledInput=DiscIntNeverNeededParam
  Ki : Gain  Gain=KiVoltage
  Kp : Gain  Gain=KpVoltage
  Sum7 : Sum  Inputs=|++
  u : Outport  VectorParamsAs1DForOutWhenUnconnected=off
  wires:
  e/1 -> Ki/1, Kp/1
  Ki/1 -> Discrete-Time Integrator/1
  Sum7/1 -> u/1
  Kp/1 -> Sum7/1
  Discrete-Time Integrator/1 -> Sum7/2
  Reset/1 -> Discrete-Time Integrator/2
